simulink model "autotune"  (R2019a)
settings: Solver=VariableStepAuto  StartTime=0.0  StopTime=10.0  RelTol=1e-3
libraries: audiosources x1, dspsnks4 x1, dspvision x1
settings Model: Creator=maddiebriere  LastModifiedBy=maddiebriere
settings DataIOCC: ReturnWorkspaceOutputs=off
settings DebuggingCC: ArithmeticOperatorsInVariantConditions=warning

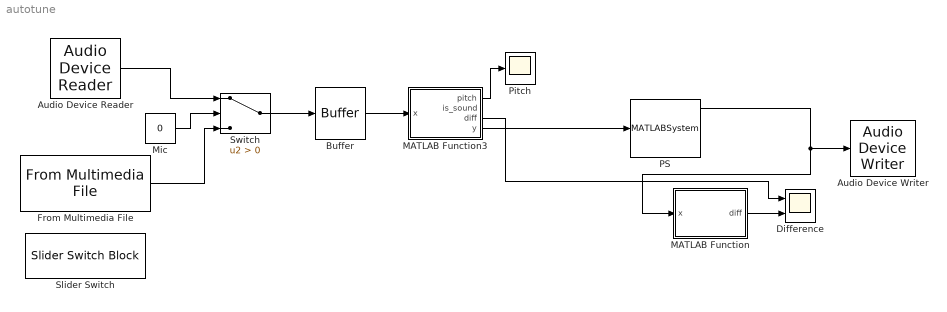
== system autotune ==
  Audio Device Reader : audiosources/Audio Device Reader  Driver=CoreAudio  Device=Default  SampleRate=44100  NumChannels=1  SamplesPerFrame=1024  BitDepth=16-bit integer  NumBuffers=10  DefaultInputChannelMapping=on  InputChannelMapping=1:2  OutputNumOverrunSamples=off  OutputDataType=double  DriverIdx=5  DeviceWarnFlag=''
      settings: SourceProductName=Audio Toolbox  SourceProductBaseCode=AU
  Audio Device Writer : dspsnks4/Audio Device Writer  Driver=CoreAudio  Device=Default  InheritSampleRate=on  SampleRate=44100  BitDepth=16-bit integer  BufferSize=4096  NumBuffers=10  DefaultOutputChannelMapping=on  OutputChannelMapping=1:2  OutputNumUnderrunSamples=off  DriverIdx=5  DeviceWarnFlag=''
  Buffer : Buffer  N=4000  OutputFrames=off
  Difference : Scope  NumInputPorts=2
  From Multimedia File : dspvision/From Multimedia File  inputFilename=/Users/maddiebriere/Desktop/Classes/8_Spring 2019/ECE485/ECE485/ECE485Labs/Final/singing44.wav  readRange=[1 Inf]  loop=on  numPlays=inf  outputStreams=Audio only  videoDataType=single  audioDataType=double  inheritSampleTime=on  userDefinedSampleTime=1/30  noAudioOutput=off  isIntensityVideo=off  fourcc=RGB  colorVideoFormat=Separate color signals  outputEOF=off  dataOrg=Column-major  audioFrameSize=1024  computeAudioFrameSize=off  outSamplingMode=Sample based
      settings: SourceProductName=DSP System Toolbox  SourceProductBaseCode=DS
  MATLAB Function : MATLAB Function  TreatAsAtomicUnit=on
  MATLAB Function3 : MATLAB Function  TreatAsAtomicUnit=on
  Mic : Constant  Value=0
  PS : MATLABSystem  System=PitchShifter  PitchShift=0  Overlap=0.01  SimulateUsing=Code generation
      mask Type: PitchShifter
      mask Display:
      | disp('PitchShifter');
      | port_label('input',1,'u');
      | port_label('output',1,'y');
      | port_label('output',2,'delays');
      | port_label('output',3,'gains');
  "Pitch " : Scope
  Slider Switch : SliderSwitchBlock
      settings: Values={{'Off', 'On'}, [0 1]}
  Switch : Switch  Criteria=u2 > Threshold
  wires:
  PS/1 -> MATLAB Function/1(x), Audio Device Writer/1
  MATLAB Function/1(diff) -> Difference/2
  MATLAB Function3/3(diff) -> Difference/1
  Buffer/1 -> MATLAB Function3/1(x)
  Audio Device Reader/1 -> Switch/1
  From Multimedia File/1 -> Switch/3
  Switch/1 -> Buffer/1
  Mic/1 -> Switch/2
  MATLAB Function3/1(pitch) -> "Pitch "/1
  MATLAB Function3/4(y) -> PS/1

== matlab function autotune/MATLAB Function ==
  data: x input; diff output
function diff = fcn(x)
[~, ~, diff] = autotune_fcn(x);
end

== matlab function autotune/MATLAB Function3 ==
  data: x input; pitch output; is_sound output; diff output; y output
function [pitch, is_sound, diff, y] = fcn(x)
[pitch, is_sound, diff] = autotune_fcn(x);
coder.extrinsic('set_param')
coder.extrinsic('num2str')
set_param('autotune/PS', 'PitchShift', num2str(diff));
y = x;
end
